simulink model "dspsacomp"  (Simulink 6.0)
settings: Solver=FixedStepDiscrete  StartTime=0.0  StopTime=inf  RelTol=1e-3  AbsTol=1e-6
libraries: dspspect3 x4, dsparch4 x1, simulink x1, dspsnks4 x1, dspsrcs4 x1
settings Model: RequirementInfo=9  Creator=don  LastModifiedBy=sconahan  ExtModeTrigMode=oneshot  ExtModeArmWhenConnect=off  BufferReuse=off  ProdHWDeviceType=Specified
settings DataIOCC: LimitDataPoints=off  SaveOutput=off  SaveTime=off  SignalLoggingName=sigsOut
settings OptimizationCC: BlockReduction=off  BooleanDataType=off  InlineInvariantSignals=off  OptimizeBlockIOStorage=off  BufferReuse=off  LocalBlockOutputs=off  MultiInstanced=off  RollThreshold=2
settings FormatCC: IgnoreBidirectionalLines=off
settings DebuggingCC: IntegerOverflowMsg=none
settings HardwareCC: ProdHWDeviceType=Specified
settings CodeAppCC: FileBanners=off  CustomSymbols=off
settings GRTTargetCC: TargetFcnLib=iso_c_tmw.mat  IsERTTarget=off

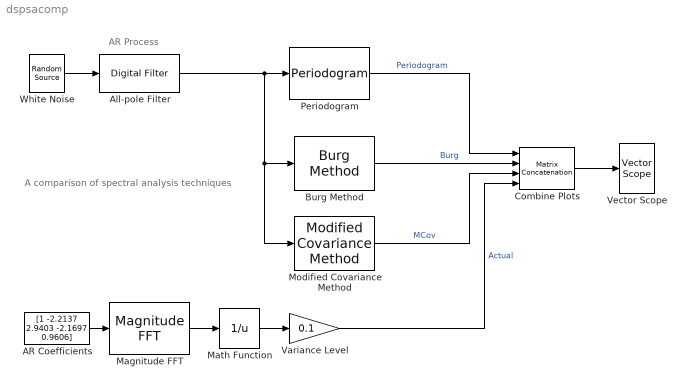
== system dspsacomp ==
  note: A comparison of spectral
      | analysis techniques
  note: AR Process
  AR Coefficients : Constant  Value=[1 -2.2137 2.9403 -2.1697 0.9606]
  All-pole Filter : dsparch4/Digital Filter  TypePopup=IIR (all poles)  IIRFiltStruct=Direct form II transposed  AllPoleFiltStruct=Direct form  FIRFiltStruct=Direct form  CoeffSource=Specify via dialog  NumCoeffs=[1 2]  DenCoeffs=[1 -2.2137 2.9403 -2.1697 0.9606]  BiQuadCoeffs=[1 0.3 0.4 1 0.1 0.2]  LatticeCoeffs=[0.2 0.4]  denIgnore=on  FiltPerSampPopup=One filter per frame  IC=0  ICnum=0  ICden=0  roundingMode=Floor  overflowMode=off
  Burg Method : dspspect3/Burg Method  inheritOrd=off  ord=4  inheritFFT=off  fftsize=128
  Combine Plots : simulink/Math Operations/Matrix Concatenation  numInports=4  catMethod=Horizontal
  Magnitude FFT : dspspect3/Magnitude FFT  mag_or_magsq=Magnitude squared  fftLenInherit=off  fftsize=128
  Math Function : Math  Operator=reciprocal  SaturateOnIntegerOverflow=on
  Modified Covariance Method : dspspect3/Modified Covariance Method  ord=4  inheritFFT=off  fftsize=128
  Periodogram : dspspect3/Periodogram  wintype=Hamming  Rs=50  beta=5  winsamp=Symmetric  inheritFFT=off  fftsize=128  navg=4
  Variance Level : Gain  Gain=0.1  SaturateOnIntegerOverflow=on
  Vector Scope : dspsnks4/Vector Scope  ScopeProperties=off  Domain=Frequency  HorizSpan=1  DisplayProperties=off  AxisGrid=on  Memory=off  FrameNumber=on  AxisLegend=on  AxisZoom=off  OpenScopeAtSimStart=on  OpenScopeImmediately=off  FigPos=[38 195 560 293]  AxisProperties=on  XUnits=Hertz  XRange=[0...Fs/2]  InheritXIncr=off  XIncr=1/1000  XLabel=Samples  YUnits=dB  YLabel=Amplitude  LineProperties=off  LineColors=[1 0 0]|[0 1 0]|[0 0 1]
      settings: YMin=-36.5241171110829  YMax=35.1414095795369
  White Noise : dspsrcs4/Random Source  SrcType=Gaussian  NormMethod=Ziggurat  CltLength=12  Min=0  Max=1  Mean=0  Var=0.1  RepMode=Specify seed  Seed=0  Inherit=off  SampMode=Discrete  SampTime=1/1000  SampFrame=64  DataType=Double  OutComplex=Real
  wires:
  White Noise/1 -> All-pole Filter/1
  Magnitude FFT/1 -> Math Function/1
  AR Coefficients/1 -> Magnitude FFT/1
  All-pole Filter/1 -> Periodogram/1, Burg Method/1, Modified Covariance Method/1
  Math Function/1 -> Variance Level/1
  Periodogram/1 -> Combine Plots/1  "Periodogram"
  Modified Covariance Method/1 -> Combine Plots/3  "MCov"
  Burg Method/1 -> Combine Plots/2  "Burg"
  Variance Level/1 -> Combine Plots/4  "Actual"
  Combine Plots/1 -> Vector Scope/1
